simulink model "lab2"  (Simulink 6.3)
settings: Solver=ode45  StartTime=0.0  StopTime=100  RelTol=1e-3
settings Model: LastModifiedBy=thill

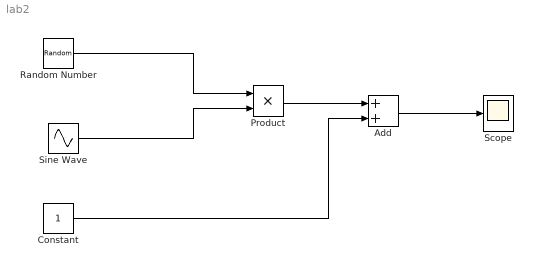
== system lab2 ==
  Add : Sum  OutScaling=2^-10
  Constant : Constant
  Product : Product  RndMeth=Zero
  Random Number : RandomNumber  SampleTime=0
  Scope : Scope
  Sine Wave : Sin  SampleTime=0
  wires:
  Sine Wave/1 -> Product/2
  Product/1 -> Add/1
  Random Number/1 -> Product/1
  Constant/1 -> Add/2
  Add/1 -> Scope/1
